simulink model "fox_bunny"  (R2022b)
settings: Solver=VariableStepAuto  StartTime=0.0  StopTime=25  FixedStep=0.001  RelTol=1e-6
settings Model: Creator=user  LastModifiedBy=user

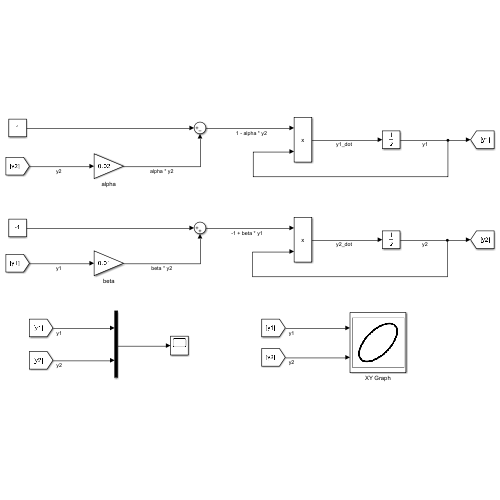
[thumbnail: Simulink's stored preview of the top-level diagram]
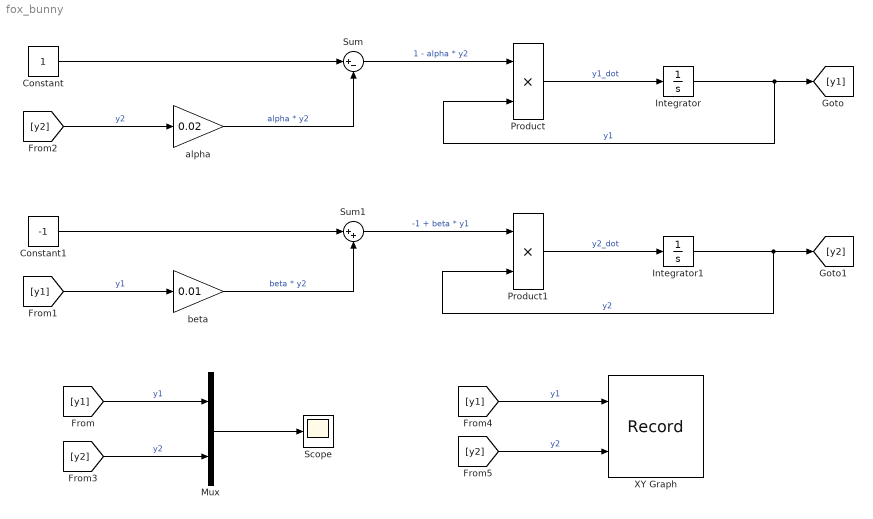
== system fox_bunny ==
  Constant : Constant
  Constant1 : Constant  Value=-1
  Integrator : Integrator  InitialCondition=20
  Integrator1 : Integrator  InitialCondition=20
  Mux : Mux  Inputs=2
  Product : Product
  Product1 : Product
  Scope : Scope
  Sum : Sum  Inputs=|+-
  Sum1 : Sum  Inputs=|++
  XY Graph : Record  FileSettingsInternal="{\"entries\":[{\"content\":{\"excelSettings\":{\"content\":{},\"type\":\"Streamout.ExcelSettings\"}},\"type\":\"Streamout.FileSettingStorage\",\"uuid\":\"\"}],\"packageUris\":[\"http:\\/\\/schema.mathworks.com\\/mf0\\/streamout_blocks\\/R2020a\"],\"version\":\"1.0\"}"  Layout=[1 1]  SignalsInternal="{\"entries\":[{\"content\":{\"signals\":[{\"content\":{\"blockPath\":[],\"channel\":[],\"dimensions\":[1],\"domain\":\"\",\"lineColor\":\"#a2142f\",\"plots\":[1],\"port\":1,\"sid\":[\"\"],\"signalID\":295,\"signalName\":\"y1\"},\"type\":\"RecordBlkView.Signal\",\"uuid\":\"\"},{\"content\":{\"blockPath\":[],\"channel\":[],\"dimensions\":[1],\"domain\":\"\",\"lineColor\":\"#139fff\",\"plots\":[1],\"port\":2,\"sid\":[\"\"],\"signalID\":299,\"signalName\":\"y2\"},\"type\":\"RecordBlkView.Signal\",\"uuid\":\"\"}]},\"type\":\"RecordBlkView.InputSignals\",\"uuid\":\"\"}],\"packageUris\":[\"http:\\/\\/schema.mathworks.com\\/mf0\\/streamout_blocks\\/R2020a\"],\"version\":\"1.0\"}"  VisualizationBindings="{\"xyplotplugin\":{\"info\":[{\"series\":[{\"bindingParametersList\":[{\"parameter\":\"X-Axis\",\"signalID\":295,\"signalName\":\"y1\"},{\"parameter\":\"Y-Axis\",\"signalID\":299,\"signalName\":\"y2\"}],\"seriesID\":22187}],\"subplotID\":1}]}}"  CompatibilityTag=XY
  alpha : Gain  Gain=0.02
  beta : Gain  Gain=0.01
  wires:
  Constant/1 -> Sum/1
  alpha/1 -> Sum/2  "alpha * y2"
  [y2] -> alpha/1  "y2"
  Sum/1 -> Product/1  "1 - alpha * y2"
  Product/1 -> Integrator/1  "y1_dot"
  Integrator/1 -> Product/2, [y1]  "y1"
  [y1] -> beta/1  "y1"
  Constant1/1 -> Sum1/1
  beta/1 -> Sum1/2  "beta * y2"
  Sum1/1 -> Product1/1  "-1 + beta * y1"
  Product1/1 -> Integrator1/1  "y2_dot"
  Integrator1/1 -> Product1/2, [y2]  "y2"
  [y1] -> Mux/1  "y1"
  [y2] -> Mux/2  "y2"
  Mux/1 -> Scope/1
  [y2] -> XY Graph/2  "y2"
  [y1] -> XY Graph/1  "y1"
